simulink model "IK_sgl_Test_speedLoop"  (R2021b)
settings: Solver=FixedStepAuto  StartTime=0.0  StopTime=600  FixedStep=0.004  RelTol=1e-3  EnableMultiTasking=on
libraries: simulink_extras x1, raspberrypiNetworklib x1
settings Model: Creator=The MathWorks, Inc.  LastModifiedBy=kboxi
settings SolverCC: ConcurrentTasks=on  AlgebraicLoopSolver=TrustRegion  PositivePriorityOrder=on
settings OptimizationCC: EnhancedBackFolding=on  PassReuseOutputArgsThreshold=0  MaxStackSize=64  OptimizeBlockOrder=speed  DifferentSizesBufferReuse=on  OptimizationCustomize=off
settings DebuggingCC: ParameterTunabilityLossMsg=error  SFMachineParentedDataDiag=warning
settings HardwareCC: ProdBitPerPointer=32  ProdBitPerSizeT=32  ProdBitPerPtrDiffT=32  ProdLargestAtomicInteger=Long  ProdLargestAtomicFloat=Double  ProdWordSize=32  ProdLongLongMode=on  ProdHWDeviceType=ARM Compatible->ARM Cortex  UseEmbeddedCoderFeatures=off
settings RTWCC: Description=Embedded Coder  SystemTargetFile=ert.tlc  HardwareBoard=Raspberry Pi  TLCOptions="-aInlineSetEventsForThisBaseRateFcn=TLC_FALSE -aSuppressMultiTaskScheduler=TLC_FALSE  -aRateBasedStepFcn=0"  TemplateMakefile=ert_default_tmf  Toolchain=GNU GCC Embedded Linux  BuildConfiguration=Faster Runs
settings CodeAppCC: ForceParamTrailComments=on  OperatorAnnotations=on
settings ERTTargetCC: ERTCustomFileBanners=off  SupportContinuousTime=on  SupportNonInlinedSFcns=on  RemoveResetFunc=off  SupportVariableSizeSignals=on  ModelStepFunctionPrototypeControlCompliant=off  ExtModeTransport=2  ExtModeStaticAlloc=on  ExtModeMexFile=ext_xcp  ExtModeIntrfLevel=Level2 - Open

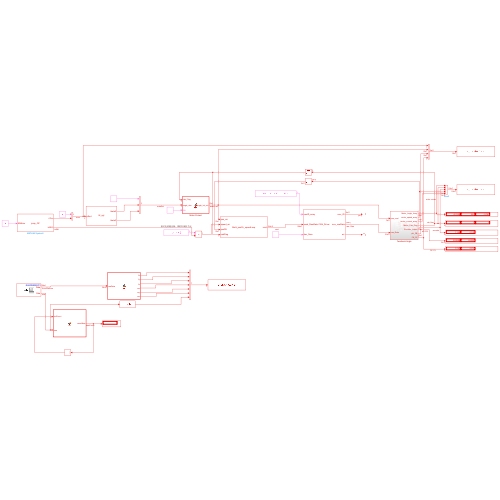
[thumbnail: Simulink's stored preview of the top-level diagram]
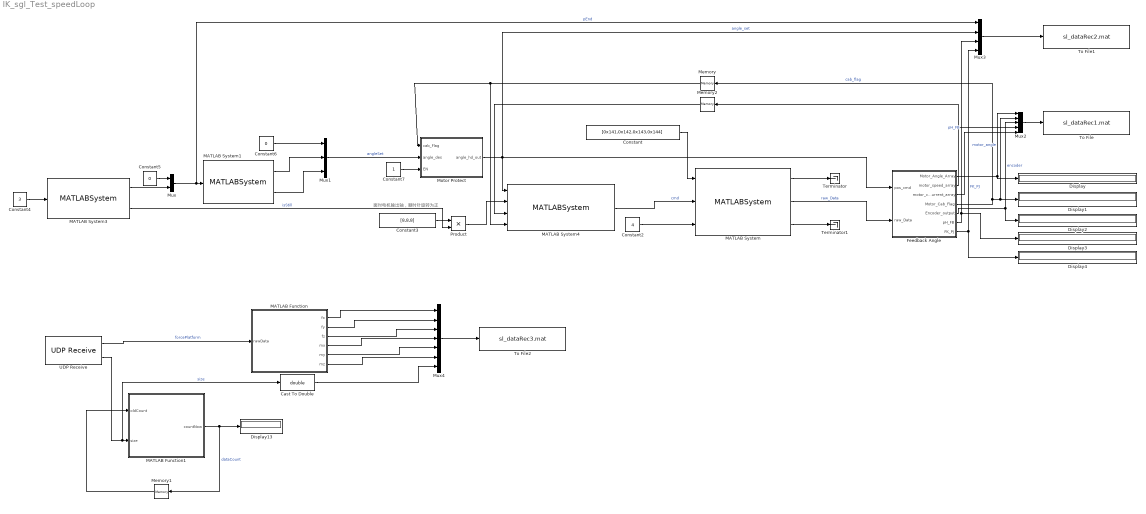
== system IK_sgl_Test_speedLoop ==
  note: 面对电机输出轴，顺时针旋转为正
  Cast To Double : DataTypeConversion  OutDataTypeStr=double
  Constant : Constant  Value=[0x141,0x142,0x143,0x144]
  Constant2 : Constant  Value=4  OutDataTypeStr=int32
  Constant3 : Constant  Value=[8,8,8]
  Constant4 : Constant  Value=3
  Constant5 : Constant  Value=0
  Constant6 : Constant  Value=0  OutDataTypeStr=double
  Constant7 : Constant
  Display{,1..4,13} (6 alike) : Display
  Feedback Angle : Subsystem
  MATLAB Function : MATLAB Function  TreatAsAtomicUnit=on
  MATLAB Function1 : MATLAB Function  TreatAsAtomicUnit=on
  MATLAB System : MATLABSystem  System=canSendRecv  canPort=can1
      mask Type: canSendRecv
      mask Display:
      | disp('CAN_Driver');
      | port_label('input',1,'canID_array');
      | port_label('input',2,'send_RawData');
      | port_label('input',3,'dev_Num');
      | port_label('output',1,'recv_ID');
      | port_label('output',2,'recv_rawData');
      | port_label('output',3,'err');
  MATLAB System1 : MATLABSystem  System=IK_sgl  SimulateUsing=Code generation
      mask Type: IK_sgl
      mask Display:
      | disp('IK_sgl');
      | port_label('input',1,'pEnd');
      | port_label('output',1,'theta2');
      | port_label('output',2,'theta3');
  MATLAB System3 : MATLABSystem  System=jump_OP  tUp=1  tDown=0.04  Amp=0.06  AmpOff=-0.5  SampleTime=0.004  OffsetTime=0  TickTime=0  SimulateUsing=Code generation
      mask Type: jump_OP
      mask Display:
      | disp('jump_OP');
      | port_label('input',1,'ENNum');
      | port_label('output',1,'zTra');
      | port_label('output',2,'isStill');
  MATLAB System4 : MATLABSystem  System=Multi_posCtr_speedLoop  dt=0.004  k_errPos=0  SimulateUsing=Code generation
      mask Type: Multi_posCtr_speedLoop
      mask Display:
      | disp('Multi_posCtr_speedLoop');
      | port_label('input',1,'pos_arr');
      | port_label('input',2,'speed_arr');
      | port_label('input',3,'posFB');
      | port_label('input',4,'cabFlag');
      | port_label('output',1,'cmd');
  Memory : Memory  InitialCondition=[0;0;0]
  Memory1 : Memory
  Memory2 : Memory  InitialCondition=[0;0;0]
  Motor Protect : MATLAB Function  TreatAsAtomicUnit=on
  Mux : Mux  Inputs=2
  Mux1 : Mux  Inputs=3
  Mux2 : Mux  Inputs=5
  Mux3 : Mux
  Mux4 : Mux  Inputs=7
  Product : Product
  Terminator : Terminator
  Terminator1 : Terminator
  To File : ToFile  Filename=sl_dataRec1.mat  MatrixName=MotorAngle_cab_Encoder_motorSpeed_motorCurrent
  To File1 : ToFile  Filename=sl_dataRec2.mat  MatrixName=pEnd_AngleSegDeg_pHFB_FKPJ
  To File2 : ToFile  Filename=sl_dataRec3.mat  MatrixName=fx_fy_fz_mx_my_mz_size
  UDP Receive : raspberrypiNetworklib/UDP Receive  localURL='0.0.0.0'  localPort=25000  remoteURL='0.0.0.0'  remotePort=-1  recvBufferSize=8192  signalDatatype=uint8  dims=24  isVarSize=off  showBlockingTime=off  blockingTime=0  sampletime=0.004  blockPlatform=Raspberry Pi
      settings: SourceProductBaseCode=RASPPI
  wires:
  Constant/1 -> MATLAB System/1
  MATLAB System4/1 -> MATLAB System/2  "cmd"
  Constant2/1 -> MATLAB System/3
  MATLAB System/1 -> Terminator/1
  MATLAB System/3 -> Terminator1/1
  MATLAB System/2 -> Feedback Angle/2(raw_Data)  "raw_Data"
  Constant4/1 -> MATLAB System3/1
  MATLAB System3/1 -> Mux/2
  Constant5/1 -> Mux/1
  Mux/1 -> Mux3/1, MATLAB System1/1  "pEnd"
  Constant6/1 -> Mux1/1
  MATLAB System1/1 -> Mux1/2
  MATLAB System1/2 -> Mux1/3
  Motor Protect/1(angle_hd_out) -> MATLAB System4/1, Feedback Angle/1(pos_cmd), Mux3/2  "angle_set"
  Constant7/1 -> Motor Protect/3(EN)
  Mux1/1 -> Motor Protect/2(angle_des)  "angleSet"
  Feedback Angle/1(Motor_Angle_Array) -> Mux2/1, Display/1  "motor_angle"
  Feedback Angle/4(Motor_Cab_Flag) -> Memory/1, Mux2/2, Display1/1  "cab_flag"
  Feedback Angle/5(Encoder_output) -> Mux2/3, Display2/1  "encoder"
  Memory/1 -> Motor Protect/1(cab_Flag), MATLAB System4/4
  Constant3/1 -> Product/1
  Product/1 -> MATLAB System4/2
  MATLAB System3/2 -> Product/2  "isStill"
  Mux2/1 -> To File/1
  Mux3/1 -> To File1/1
  Feedback Angle/6(pH_FB) -> Mux3/3, Display3/1  "pH_FB"
  Feedback Angle/7(FK_PJ) -> Mux3/4, Display4/1  "FK_PJ"
  UDP Receive/1 -> MATLAB Function/1(rawData)  "forcePlatform"
  UDP Receive/2 -> Cast To Double/1, MATLAB Function1/2(size)  "size"
  MATLAB Function/1(fx) -> Mux4/1
  MATLAB Function/2(fy) -> Mux4/2
  MATLAB Function/3(fz) -> Mux4/3
  MATLAB Function/4(mx) -> Mux4/4
  MATLAB Function/5(my) -> Mux4/5
  MATLAB Function/6(mz) -> Mux4/6
  MATLAB Function1/1(countNow) -> Memory1/1, Display13/1  "dataCount"
  Memory1/1 -> MATLAB Function1/1(oldCount)
  Mux4/1 -> To File2/1
  Cast To Double/1 -> Mux4/7
  Feedback Angle/2(motor_speed_array) -> Memory2/1, Mux2/4
  Feedback Angle/3(motor_current_array) -> Mux2/5
  Memory2/1 -> MATLAB System4/3

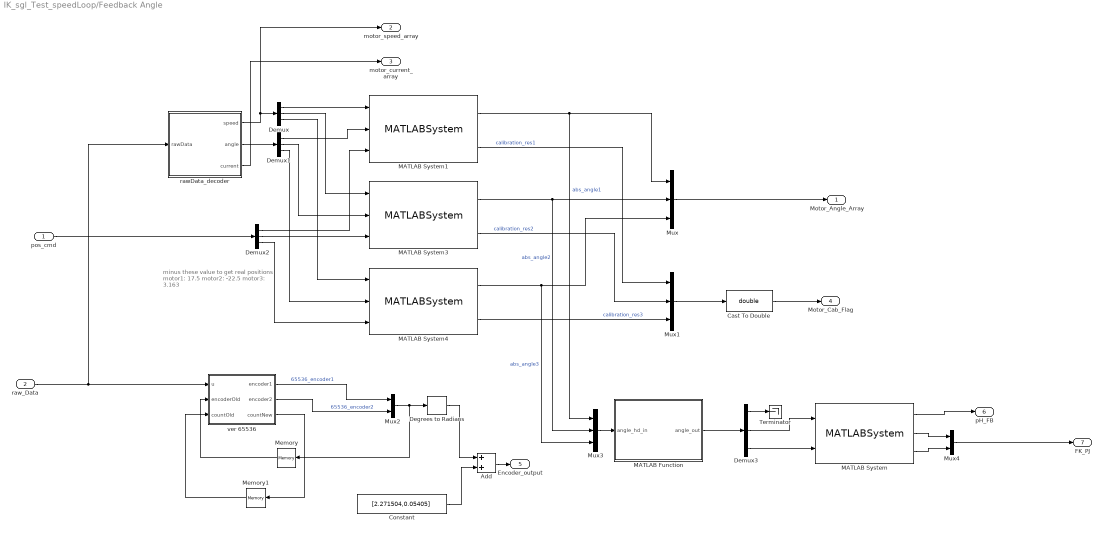
== system IK_sgl_Test_speedLoop/Feedback Angle ==
  note: minus these value to get real positions
      | motor1: 17.5
      | motor2: -22.5
      | motor3: 3.163
  pos_cmd : Inport
  raw_Data : Inport  Port=2
  Add : Sum
  Cast To Double : DataTypeConversion  OutDataTypeStr=double
  Constant : Constant  Value=[2.271504,0.05405]
  Degrees to Radians : simulink_extras/Transformations/Degrees to Radians
  Demux{,1..3} (4 alike) : Demux  Outputs=3
  MATLAB Function : MATLAB Function  TreatAsAtomicUnit=on
  MATLAB System : MATLABSystem  System=FK_sgl  SimulateUsing=Code generation
      mask Type: FK_sgl
      mask Display:
      | disp('FK_sgl');
      | port_label('input',1,'theta2');
      | port_label('input',2,'theta3');
      | port_label('output',1,'pH');
      | port_label('output',2,'BDG');
      | port_label('output',3,'DGH');
  MATLAB System1 : MATLABSystem  System=MotorAngle  angleOff=-17.5  SimulateUsing=Code generation
      mask Type: MotorAngle
      mask Display:
      | disp('MotorAngle');
      | port_label('input',1,'speed');
      | port_label('input',2,'sgl_angle');
      | port_label('input',3,'pos_des');
      | port_label('output',1,'abs_angle');
      | port_label('output',2,'calibration');
  MATLAB System3 : MATLABSystem  System=MotorAngle  angleOff=22.5  SimulateUsing=Code generation
      mask Type: MotorAngle
      mask Display:
      | disp('MotorAngle');
      | port_label('input',1,'speed');
      | port_label('input',2,'sgl_angle');
      | port_label('input',3,'pos_des');
      | port_label('output',1,'abs_angle');
      | port_label('output',2,'calibration');
  MATLAB System4 : MATLABSystem  System=MotorAngle  angleOff=-3.163  SimulateUsing=Code generation
      mask Type: MotorAngle
      mask Display:
      | disp('MotorAngle');
      | port_label('input',1,'speed');
      | port_label('input',2,'sgl_angle');
      | port_label('input',3,'pos_des');
      | port_label('output',1,'abs_angle');
      | port_label('output',2,'calibration');
  Memory : Memory  InitialCondition=[999;999]
  Memory1 : Memory
  Mux : Mux  Inputs=3
  Mux1 : Mux  Inputs=3
  Mux2 : Mux  Inputs=2
  Mux3 : Mux  Inputs=3
  Mux4 : Mux  Inputs=2
  Terminator : Terminator
  rawData_decoder : MATLAB Function  TreatAsAtomicUnit=on
  ver 65536 : MATLAB Function  TreatAsAtomicUnit=on
  Motor_Angle_Array : Outport
  motor_speed_array : Outport  Port=2
  motor_current_array : Outport  Port=3
  Motor_Cab_Flag : Outport  Port=4
  Encoder_output : Outport  Port=5
  pH_FB : Outport  Port=6
  FK_PJ : Outport  Port=7
  wires:
  Demux/3 -> MATLAB System4/1
  raw_Data/1 -> ver 65536/1(u), rawData_decoder/1(rawData)
  MATLAB System3/1 -> Mux3/2, Mux/2  "abs_angle2"
  Demux1/1 -> MATLAB System1/2
  rawData_decoder/1(speed) -> motor_speed_array/1, Demux/1
  MATLAB System1/1 -> Mux/1, Mux3/1  "abs_angle1"
  ver 65536/2(encoder2) -> Mux2/2  "65536_encoder2"
  rawData_decoder/2(angle) -> Demux1/1
  Demux/1 -> MATLAB System1/1
  Demux1/2 -> MATLAB System3/2
  MATLAB System1/2 -> Mux1/1  "calibration_res1"
  pos_cmd/1 -> Demux2/1
  MATLAB System4/2 -> Mux1/3  "calibration_res3"
  MATLAB System3/2 -> Mux1/2  "calibration_res2"
  Demux1/3 -> MATLAB System4/2
  Demux2/2 -> MATLAB System3/3
  Demux/2 -> MATLAB System3/1
  Demux2/3 -> MATLAB System4/3
  ver 65536/1(encoder1) -> Mux2/1  "65536_encoder1"
  Demux2/1 -> MATLAB System1/3
  MATLAB System4/1 -> Mux/3, Mux3/3  "abs_angle3"
  Mux/1 -> Motor_Angle_Array/1
  Mux3/1 -> MATLAB Function/1(angle_hd_in)
  MATLAB Function/1(angle_out) -> Demux3/1
  Demux3/2 -> MATLAB System/1
  Demux3/3 -> MATLAB System/2
  Demux3/1 -> Terminator/1
  MATLAB System/1 -> pH_FB/1
  MATLAB System/3 -> Mux4/2
  MATLAB System/2 -> Mux4/1
  Mux4/1 -> FK_PJ/1
  Mux2/1 -> Memory/1, Degrees to Radians/1
  Mux1/1 -> Cast To Double/1
  Cast To Double/1 -> Motor_Cab_Flag/1
  Constant/1 -> Add/2
  Degrees to Radians/1 -> Add/1
  Add/1 -> Encoder_output/1
  Memory/1 -> ver 65536/2(encoderOld)
  ver 65536/3(countNew) -> Memory1/1
  Memory1/1 -> ver 65536/3(countOld)
  rawData_decoder/3(current) -> motor_current_array/1

== matlab function IK_sgl_Test_speedLoop/Feedback Angle/ver 65536 ==
  data: u input uint8 size=[32,1]; encoder1 output double size=[1,1]; encoder2 output double size=[1,1]; encoderOld input size=[2,1]; countOld input size=[1,1]; countNew output size=[1,1]
function [encoder1,encoder2,countNew] = fcn(u,encoderOld,countOld)
rowEnd=u(25:32);
encoder2=-double(typecast(rowEnd(1:2),'uint16'))/65536*360;
encoder1=-double(typecast(rowEnd(3:4),'uint16'))/65536*360;
if countOld<1000
    countNew=countOld+1;
    return;
else
    countNew=countOld;
end
if abs(encoder1-encoderOld(1))>10
    encoder1=encoderOld(1);
end
if abs(encoder2-encoderOld(2))>10
    encoder2=encoderOld(2);
end

== matlab function IK_sgl_Test_speedLoop/Motor Protect ==
  data: cab_Flag input; angle_hd_out output; angle_des input; EN input
function angle_hd_out = fcn(cab_Flag,angle_des,EN)
if sum(cab_Flag)<2.5
    angle_hd_out=[0;0;0];
else
    if EN>0.5
        angle_hd_out=angle_des/pi*180*(-1);
    else
        angle_hd_out=[0;0;0];
    end
end
if angle_hd_out(1)>10
    angle_hd_out(1)=10;
end
if angle_hd_out(1)<-10
    angle_hd_out(1)=-10;
end
if angle_hd_out(2)>30
    angle_hd_out(2)=30;
end
if angle_hd_out(2)<-10
    angle_hd_out(2)=-10;
end
if angle_hd_out(3)>45
    angle_hd_out(3)=45;
end
if angle_hd_out(3)<-25
    angle_hd_out(3)=-25;
end

== matlab function IK_sgl_Test_speedLoop/Feedback Angle/rawData_decoder ==
  data: speed output; rawData input uint8; angle output; current output
function [speed,angle,current] = fcn(rawData)
% angle : single loop position, degree
% speed : speed after the reducer, degree per second
angle=zeros(3,1);
speed=zeros(3,1);
current=zeros(3,1);
for i=1:1:3
    idx=i*8-7;
    angle(i) = double(typecast(rawData(idx+6:idx+7),'uint16'))/65535*360;
    speed(i) = double(typecast(rawData(idx+4:idx+5),'int16'))/6;
    current(i) = double(typecast(rawData(idx+2:idx+3),'int16'));
end

== matlab function IK_sgl_Test_speedLoop/Feedback Angle/MATLAB Function ==
  data: angle_hd_in input; angle_out output
function angle_out = fcn(angle_hd_in)
angle_out=angle_hd_in/180*pi*(-1);

== matlab function IK_sgl_Test_speedLoop/MATLAB Function ==
  data: rawData input; fx output size=[1,1]; fy output size=[1,1]; fz output size=[1,1]; mx output size=[1,1]; my output size=[1,1]; mz output size=[1,1]
function [fx,fy,fz,mx,my,mz] = fcn(rawData)
% angle : single loop position, degree
% speed : speed after the reducer, degree per second
fx=double(typecast(rawData(1:4),'single'));
fy=double(typecast(rawData(5:8),'single'));
fz=double(typecast(rawData(9:12),'single'));
mx=double(typecast(rawData(13:16),'single'));
my=double(typecast(rawData(17:20),'single'));
mz=double(typecast(rawData(21:24),'single'));

== matlab function IK_sgl_Test_speedLoop/MATLAB Function1 ==
  data: oldCount input; countNow output size=[1,1]; size input
function countNow = fcn(oldCount,size)
% angle : single loop position, degree
% speed : speed after the reducer, degree per second
if size>23
    countNow=oldCount+1;
else
    countNow=oldCount;
end
